simulink model "STanque01"  (R2013a)
settings: Solver=ode45  StartTime=0.0  StopTime=1000  RelTol=1e-3
settings Model: Creator=Cristhian Ivan  LastModifiedBy=Cristhian Ivan

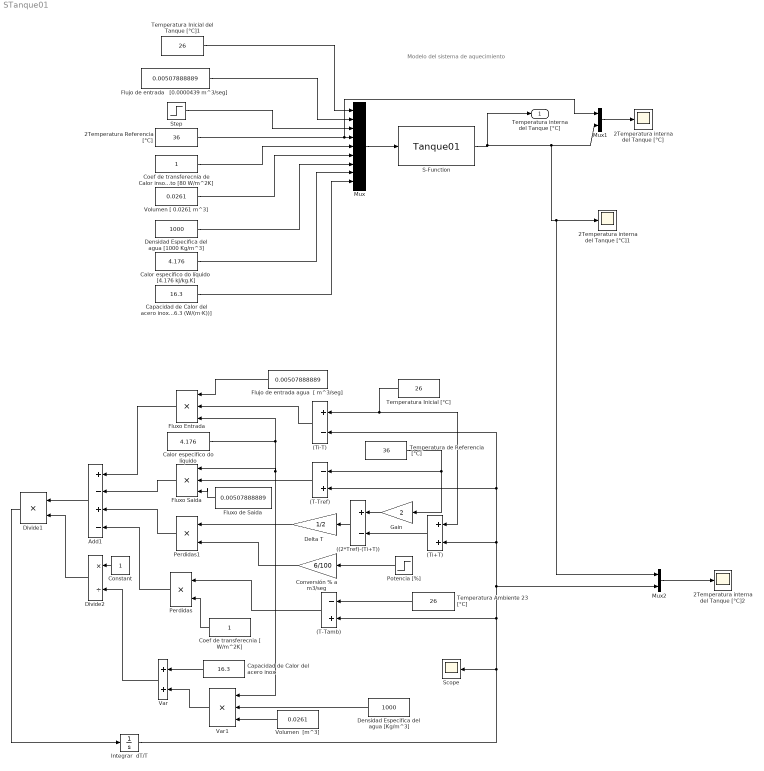
== system STanque01 ==
  note: Modelo del sistema de aquecimiento
  ((2*Tref)-(Ti+T)) : Sum  Inputs=+-
  (T-Tamb) : Sum  Inputs=-+
  (T-Tref) : Sum  Inputs=-+
  (Ti+T) : Sum
  (Ti-T) : Sum  Inputs=+-
  2Temperatura Referencia [°C] : Constant  Value=36
  2Temperatura interna del Tanque [°C] : Scope
      settings: TimeRange=10  YMin=20  YMax=45
  2Temperatura interna del Tanque [°C]1 : Scope
      settings: TimeRange=10  YMin=20  YMax=45  SaveName=RespSimulada
  2Temperatura interna del Tanque [°C]2 : Scope
      settings: TimeRange=10  YMin=20  YMax=45  SaveName=RespSimulada1
  Add1 : Sum  Inputs=+-+-
  Calor especifico do líquido : Constant  Value=4.176
  Calor especifico do líquido  [4.176 kJ/kg.K] : Constant  Value=4.176
  "Capacidad de Calor del acero inox " : Constant  Value=16.3
  Capacidad de Calor del acero inox [16.3 (W/(m·K))] : Constant  Value=16.3
  Coef de transferecnia [ W/m^2K] : Constant
  Coef de transferecnia de Calor insolamiento [80 W/m^2K] : Constant
  Constant : Constant
  Conversión % a m3/seg : Gain  Gain=6/100
  Delta T : Gain  Gain=1/2
  Densidad Especifica del agua [1000 Kg/m^3] : Constant  Value=1000
  "Densidad Especifica del agua [Kg/m^3] " : Constant  Value=1000
  Divide1 : Product  Inputs=**
  Divide2 : Product  Inputs=*/
  "Flujo de entrada   [0.0000439 m^3/seg] " : Constant  Value=0.00507888889
  Flujo de entrada agua  [ m^3/seg] : Constant  Value=0.00507888889
  Fluxo Entrada : Product  Inputs=***
  Fluxo Saida : Product  Inputs=***
  "Fluxo de Saida  " : Constant  Value=0.00507888889
  Gain : Gain  Gain=2
  Integrar  dT/T : Integrator
  Mux : Mux  Inputs=9
  Mux1 : Mux  Inputs=2
  Mux2 : Mux  Inputs=2
  Perdidas : Product  Inputs=**
  Perdidas1 : Product  Inputs=**
  Potencia [%] : Step  Time=0  After=30  SampleTime=0
  S-Function : S-Function  FunctionName=Tanque01  EnableBusSupport=off
  Scope : Scope
      settings: TimeRange=10  YMin=58.165  YMax=58.225
  Step : Step  Time=0  After=20  SampleTime=0
  "Temperatura Ambiente 23 [°C] " : Constant  Value=26
  Temperatura Inicial [°C] : Constant  Value=26
  Temperatura Inicial del Tanque [°C]1 : Constant  Value=26
  Temperatura de Referencia  [°C] : Constant  Value=36
  Var : Sum
  Var1 : Product  Inputs=***
  Volumen  [m^3] : Constant  Value=0.0261
  Volumen [ 0.0261 m^3] : Constant  Value=0.0261
  Temperatura interna del Tanque [°C] : Outport
  wires:
  Volumen [ 0.0261 m^3]/1 -> Mux/6
  Capacidad de Calor del acero inox [16.3 (W/(m·K))]/1 -> Mux/9
  Calor especifico do líquido  [4.176 kJ/kg.K]/1 -> Mux/8
  S-Function/1 -> Temperatura interna del Tanque [°C]/1, Mux2/1, 2Temperatura interna del Tanque [°C]1/1, Mux1/2
  Coef de transferecnia de Calor insolamiento [80 W/m^2K]/1 -> Mux/5
  Mux/1 -> S-Function/1
  Densidad Especifica del agua [1000 Kg/m^3]/1 -> Mux/7
  Temperatura Inicial del Tanque [°C]1/1 -> Mux/1
  "Flujo de entrada   [0.0000439 m^3/seg] "/1 -> Mux/2
  2Temperatura Referencia [°C]/1 -> Mux1/1, Mux/4
  Mux1/1 -> 2Temperatura interna del Tanque [°C]/1
  Step/1 -> Mux/3
  Add1/1 -> Divide1/1
  Fluxo Entrada/1 -> Add1/1
  Temperatura Inicial [°C]/1 -> (Ti+T)/1, (Ti-T)/1
  Calor especifico do líquido/1 -> Var1/1, Fluxo Saida/1, Fluxo Entrada/3
  "Densidad Especifica del agua [Kg/m^3] "/1 -> Var1/2
  "Capacidad de Calor del acero inox "/1 -> Var/1
  Var1/1 -> Var/2
  Volumen  [m^3]/1 -> Var1/3
  Potencia [%]/1 -> Conversión % a m3/seg/1
  Divide1/1 -> Integrar  dT/T/1
  "Fluxo de Saida  "/1 -> Fluxo Saida/3
  Flujo de entrada agua  [ m^3/seg]/1 -> Fluxo Entrada/1
  Perdidas/1 -> Add1/4
  Coef de transferecnia [ W/m^2K]/1 -> Perdidas/2
  "Temperatura Ambiente 23 [°C] "/1 -> (T-Tamb)/1
  (T-Tamb)/1 -> Perdidas/1
  Divide2/1 -> Divide1/2
  Constant/1 -> Divide2/1
  Var/1 -> Divide2/2
  (Ti-T)/1 -> Fluxo Entrada/2
  (Ti+T)/1 -> ((2*Tref)-(Ti+T))/2
  Gain/1 -> ((2*Tref)-(Ti+T))/1
  ((2*Tref)-(Ti+T))/1 -> Delta T/1
  Perdidas1/1 -> Add1/3
  Delta T/1 -> Perdidas1/1
  Conversión % a m3/seg/1 -> Perdidas1/2
  Temperatura de Referencia  [°C]/1 -> Gain/1, (T-Tref)/1
  Integrar  dT/T/1 -> (T-Tamb)/2, Mux2/2, (T-Tref)/2, (Ti-T)/2, (Ti+T)/2, Scope/1
  Mux2/1 -> 2Temperatura interna del Tanque [°C]2/1
  Fluxo Saida/1 -> Add1/2
  (T-Tref)/1 -> Fluxo Saida/2
